simulink model "SF038A_LimrCdng"  (R2013b)
settings: Solver=FixedStepDiscrete  StartTime=0.0  StopTime=1  FixedStep=.002  RelTol=1e-3
values from neighbouring files (symbols this model uses):
  ARCHGLBPRM_2MILLISEC_SEC_F32 = DataDict.Constant    [SF038A_LimrCdng_DataDict.m]
  FLTINJ_LIMRCDNG_EOTGAIN = DataDict.Constant    [SF038A_LimrCdng_DataDict.m]
  FLTINJ_LIMRCDNG_EOTLIM = DataDict.Constant    [SF038A_LimrCdng_DataDict.m]
  FLTINJ_LIMRCDNG_SYSMOTTQCMDSCA = DataDict.Constant    [SF038A_LimrCdng_DataDict.m]
  LimrCdngGainDecSlew = DataDict.Calibration    [SF038A_LimrCdng_DataDict.m]
  LimrCdngTqDecSlew = DataDict.Calibration    [SF038A_LimrCdng_DataDict.m]
libraries: NxtrLim x12, FixdToFloat x2, LnrIntrpn x2, FloatToFixd x1, simulink x1
Description:
  | This function provides a layer of protection from erroneous signals feeding into SF-04 Sum & Limit.
  | It is applied primarily to 'limiting' signals that serve to reduce motor torque command under certain
  | operating conditions.  This function can prevent step response or 'toggling' behavior that might cause
  | undesirable vehicle feel.  It includes capability of fault injection at some inputs to facilitate tuning.
settings Model: CovMetricSettings=dcmw  CovHTMLOptions=-sRT=1 -aTS=1 -bRG=1 -bTC=1 -hTR=0 -nFC=0 -scm=1 -bcm=1 -xEv=0  Creator=Kevin Derry  LastModifiedBy=bzhf94
settings Model: ModifiedHistory=|
  | 001
  | Initial release
  | Kevin Derry
  | 15-Aug-2012
  | ICR-3666
  | 
  | 002
  | Add vehicle speed dependency to rate limiter cals applied during recovery (increasing direction).
  | Rename and share cals among rate limiters.
  | Scott Millsap
  | 14-May-2013
  | ICR-4115
  | 
  | 003
  | Added new input CCL_TrqRamp_Uls, a torque scaling factor calculated in the MSA function, and a rate limiter to limit the rate at which it changes.
  | Added new calibration to adjust the decreasing slew rate for CCL_TrqRamp_Uls.
  | Prerit Pramod
  | 09-July-2013
  | ICR-4202
  | 
  | 4.0.0
  | Updated Model according to the new FDD standards and tool chain.
  | Siva
  | 04-Feb-2015
  | ICR-XXXX
settings DataIOCC: LimitDataPoints=off  SaveFormat=Structure  ReturnWorkspaceOutputs=on
settings OptimizationCC: BlockReduction=off  InlineParams=on  ZeroExternalMemoryAtStartup=off  ZeroInternalMemoryAtStartup=off  OptimizeModelRefInitCode=on  LifeSpan=1
settings DebuggingCC: SignalInfNanChecking=error  SignalRangeChecking=warning  UnderspecifiedInitializationDetection=Simplified  SolverPrmCheckMsg=error  InheritedTsInSrcMsg=error  DiscreteInheritContinuousMsg=error  SingleTaskRateTransMsg=error  TasksWithSamePriorityMsg=error  SigSpecEnsureSampleTimeMsg=error  CheckMatrixSingularityMsg=error  IntegerOverflowMsg=error  ParameterUnderflowMsg=error  ParameterPrecisionLossMsg=error  ParameterTunabilityLossMsg=error  FixptConstUnderflowMsg=warning  FixptConstOverflowMsg=warning  VectorMatrixConversionMsg=error  SignalLabelMismatchMsg=error  UnconnectedInputMsg=error  UnconnectedOutputMsg=error  UnconnectedLineMsg=error  SFcnCompatibilityMsg=error  UniqueDataStoreMsg=warning  BusObjectLabelMismatch=error  RootOutportRequireBusObject=error  AssertControl=DisableAll  ModelReferenceIOMsg=error  ModelReferenceVersionMismatchMessage=warning  ModelReferenceIOMismatchMessage=error  ModelReferenceCSMismatchMessage=warning  ModelReferenceDataLoggingMessage=error  StateNameClashWarn=warning  StrictBusMsg=ErrorOnBusTreatedAsVector  NonBusSignalsTreatedAsBus=error  SFUnexpectedBacktrackingDiag=error  SFInvalidInputDataAccessInChartInitDiag=error  SFNoUnconditionalDefaultTransitionDiag=error  SFTransitionOutsideNaturalParentDiag=error  SFUnconditionalTransitionShadowingDiag=error  SFUndirectedBroadcastEventsDiag=error
settings ModelReferenceCC: ModelReferenceNumInstancesAllowed=Single
settings RTWCC: SystemTargetFile=autosar.tlc  GenCodeOnly=on  TemplateMakefile=ert_default_tmf  Description=AUTOSAR  GenerateReport=on  ProcessScript=autosar_make_rtw_hook  LaunchReport=on
settings CodeAppCC: GenerateComments=off  IgnoreCustomStorageClasses=off  CustomSymbolStrType=$N$R$M  CustomSymbolStrBlkIO=$N$M  SimulinkBlockComments=off
settings STFCustomTargetCC: ParMdlRefBuildCompliant=on  CompOptLevelCompliant=on  IncludeMdlTerminateFcn=off  CombineOutputUpdateFcns=on  SuppressErrorStatus=on  ERTFirstTimeCompliant=on  ERTCustomFileBanners=on  SupportNonFinite=off  SupportComplex=off  SupportContinuousTime=off  SupportNonInlinedSFcns=off  MATLABClassNameForMDSCustomization=Simulink.SoftwareTarget.ERTCustomization  AutosarCompliant=on  GRTInterface=off  SystemTargetFile=autosar.tlc
settings ERTTargetCC: CodeReplacementLibrary=ANSI_C  ConcurrentExecutionCompliant=off  IncludeMdlTerminateFcn=off  SuppressErrorStatus=on  SupportNonFinite=off  SupportComplex=off  ModelStepFunctionPrototypeControlCompliant=off  CPPClassGenCompliant=off  AutosarCompliant=on  InlinedParameterPlacement=NonHierarchical  ERTCustomFileTemplate=example_file_process.tlc  EnableUserReplacementTypes=on

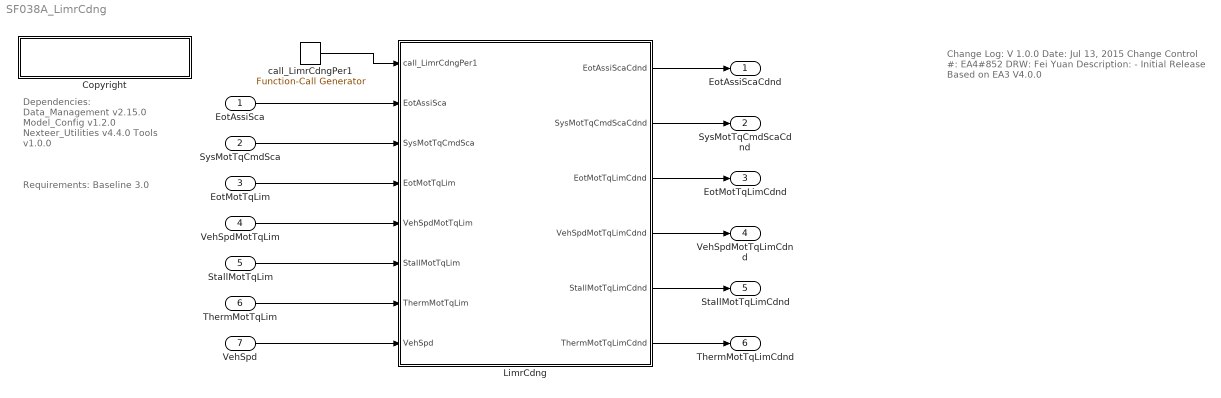
== system SF038A_LimrCdng ==
  note: Requirements: Baseline 3.0
  note: Dependencies:
      |   Data_Management v2.15.0
      |   Model_Config v1.2.0
      |   Nexteer_Utilities v4.4.0
      |   Tools v1.0.0
  note: Change Log:
      |
      | V 1.0.0
      | Date: Jul 13, 2015
      | Change Control #: EA4#852
      | DRW: Fei Yuan
      | Description:
      | - Initial Release Based on EA3 V4.0.0
  EotAssiSca : Inport
  SysMotTqCmdSca : Inport  Port=2
  EotMotTqLim : Inport  Port=3
  VehSpdMotTqLim : Inport  Port=4
  StallMotTqLim : Inport  Port=5
  ThermMotTqLim : Inport  Port=6
  VehSpd : Inport  Port=7
  Copyright : Subsystem  Description=|  mask(Copyright Information){none=on}
      | Copyright info block.                                               
      |                                                                     
      | Place copyright information at the top of every subsystem in design.
      mask prompts: none "No parameters"
      mask help: Place copyright information at the top of every subsystem in design.
      mask Display:
      | NxtrConf = 'Nexteer Confidential';
      | 
      | sys = bdroot; %handle for the current model ("system")
      | first = get_param(sys,'Created');
      | first = first(end-3:end);  %year is last four digits
      | 
      | last = get_param(sys,'LastModifiedDate');
      | if isempty(last)
      |     last = datestr(now,'yyyy');
      | else
      |     last = last(end-3:end);
      | end
      | 
      | if strcmp(first,last)
      |     fprintf('%s\nCopyright  %s Nexteer',NxtrConf,first);
      | else
      |     fprintf('%s\n%s%s-%s Nexteer',NxtrConf,char(169),first,last);
      | end
  LimrCdng : Subsystem
  call_LimrCdngPer1 : simulink/Ports & Subsystems/Function-Call Generator  RequirementInfo="{'linktype_rmi_doors' '0000a53e (/E-STEER Core/SubSystem Specifications/Application Functions/SF038A Limiter Conditioning)' '#SF038A_52' 'true' 'REQ:  SF038A_52' '' } %GIDa_33899db9_96af_4043_bf12_1f8199c4a9fb"  sample_time=0.002  numberOfIterations=1
      settings: AttributesFormatString=%<sample_time>
  EotAssiScaCdnd : Outport
  SysMotTqCmdScaCdnd : Outport  Port=2
  EotMotTqLimCdnd : Outport  Port=3
  VehSpdMotTqLimCdnd : Outport  Port=4
  StallMotTqLimCdnd : Outport  Port=5
  ThermMotTqLimCdnd : Outport  Port=6
  wires:
  call_LimrCdngPer1/1 -> LimrCdng/1(call_LimrCdngPer1)
  LimrCdng/3(EotMotTqLimCdnd) -> EotMotTqLimCdnd/1
  LimrCdng/4(VehSpdMotTqLimCdnd) -> VehSpdMotTqLimCdnd/1
  LimrCdng/5(StallMotTqLimCdnd) -> StallMotTqLimCdnd/1
  LimrCdng/6(ThermMotTqLimCdnd) -> ThermMotTqLimCdnd/1
  LimrCdng/2(SysMotTqCmdScaCdnd) -> SysMotTqCmdScaCdnd/1
  LimrCdng/1(EotAssiScaCdnd) -> EotAssiScaCdnd/1
  VehSpdMotTqLim/1 -> LimrCdng/5(VehSpdMotTqLim)
  ThermMotTqLim/1 -> LimrCdng/7(ThermMotTqLim)
  SysMotTqCmdSca/1 -> LimrCdng/3(SysMotTqCmdSca)
  EotMotTqLim/1 -> LimrCdng/4(EotMotTqLim)
  EotAssiSca/1 -> LimrCdng/2(EotAssiSca)
  StallMotTqLim/1 -> LimrCdng/6(StallMotTqLim)
  VehSpd/1 -> LimrCdng/8(VehSpd)

== system SF038A_LimrCdng/Copyright ==

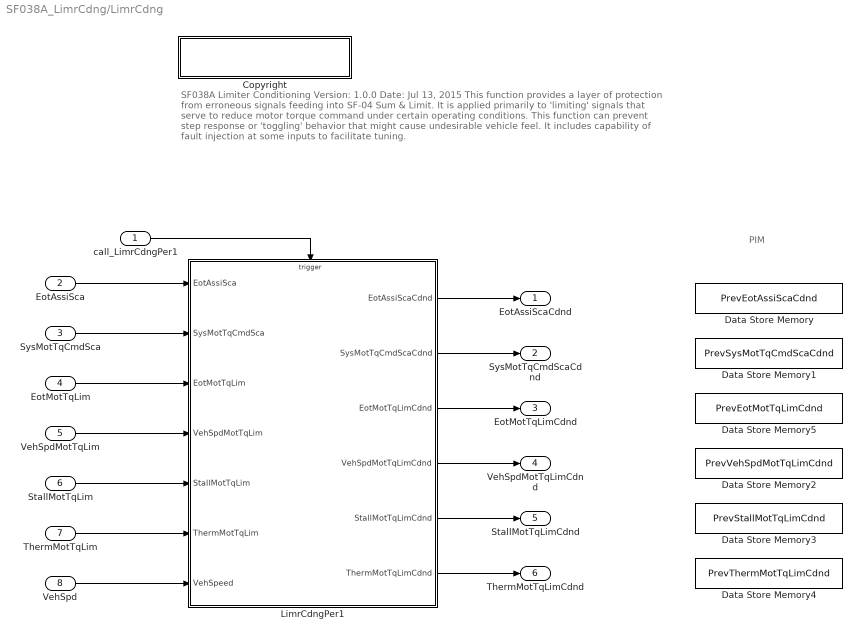
== system SF038A_LimrCdng/LimrCdng ==
  note: PIM
  note: SF038A  Limiter Conditioning
      | Version:  1.0.0     Date:  Jul 13, 2015
      |
      | This function provides a layer of protection from erroneous signals feeding into SF-04 Sum & Limit.
      | It is applied primarily to 'limiting' signals that serve to reduce motor torque command under certain
      | operating conditions.  This function can prevent step response or 'toggling' behavior that might cause
      | undesirable vehicle feel.  It includes capability of fault injection at some inputs to facilitate tuning.
  call_LimrCdngPer1 : Inport
  EotAssiSca : Inport  RequirementInfo="{'linktype_rmi_doors' '0000a53e (/E-STEER Core/SubSystem Specifications/Application Functions/SF038A Limiter Conditioning)' '#SF038A_9' 'true' 'REQ:  SF038A_9' '' } %GIDa_95b6a5c9_0ea2_4b71_a18e_8af6141b721d"  Port=2
  SysMotTqCmdSca : Inport  RequirementInfo="{'linktype_rmi_doors' '0000a53e (/E-STEER Core/SubSystem Specifications/Application Functions/SF038A Limiter Conditioning)' '#SF038A_32' 'true' 'REQ:  SF038A_32' '' } %GIDa_d644cb2e_06c7_46bd_9f8c_2e58e9e11dd4"  Port=3
  EotMotTqLim : Inport  RequirementInfo="{'linktype_rmi_doors' '0000a53e (/E-STEER Core/SubSystem Specifications/Application Functions/SF038A Limiter Conditioning)' '#SF038A_33' 'true' 'REQ:  SF038A_33' '' } %GIDa_34eaac59_c46a_4a86_98aa_7316f8ddc777"  Port=4
  VehSpdMotTqLim : Inport  RequirementInfo="{'linktype_rmi_doors' '0000a53e (/E-STEER Core/SubSystem Specifications/Application Functions/SF038A Limiter Conditioning)' '#SF038A_34' 'true' 'REQ:  SF038A_34' '' } %GIDa_5871f326_e5eb_4bf5_971f_60224a1642be"  Port=5
  StallMotTqLim : Inport  RequirementInfo="{'linktype_rmi_doors' '0000a53e (/E-STEER Core/SubSystem Specifications/Application Functions/SF038A Limiter Conditioning)' '#SF038A_35' 'true' 'REQ:  SF038A_35' '' } %GIDa_b9e54dce_09d0_4883_abfa_7d2a02c8cade"  Port=6
  ThermMotTqLim : Inport  RequirementInfo="{'linktype_rmi_doors' '0000a53e (/E-STEER Core/SubSystem Specifications/Application Functions/SF038A Limiter Conditioning)' '#SF038A_36' 'true' 'REQ:  SF038A_36' '' } %GIDa_e62a3544_49ac_4587_8d34_9b4d1dff1da3"  Port=7
  VehSpd : Inport  RequirementInfo="{'linktype_rmi_doors' '0000a53e (/E-STEER Core/SubSystem Specifications/Application Functions/SF038A Limiter Conditioning)' '#SF038A_37' 'true' 'REQ:  SF038A_37' '' } %GIDa_20705676_3852_4d53_b159_210d5e5d8ae2"  Port=8
  Copyright : Subsystem  Description=|  mask(Copyright Information){none=on}
      | Copyright info block.                                               
      |                                                                     
      | Place copyright information at the top of every subsystem in design.
      mask prompts: none "No parameters"
      mask help: Place copyright information at the top of every subsystem in design.
      mask Display:
      | NxtrConf = 'Nexteer Confidential';
      | 
      | sys = bdroot; %handle for the current model ("system")
      | first = get_param(sys,'Created');
      | first = first(end-3:end);  %year is last four digits
      | 
      | last = get_param(sys,'LastModifiedDate');
      | if isempty(last)
      |     last = datestr(now,'yyyy');
      | else
      |     last = last(end-3:end);
      | end
      | 
      | if strcmp(first,last)
      |     fprintf('%s\nCopyright  %s Nexteer',NxtrConf,first);
      | else
      |     fprintf('%s\n%s%s-%s Nexteer',NxtrConf,char(169),first,last);
      | end
  Data Store Memory : DataStoreMemory  DataStoreName=PrevEotAssiScaCdnd  StateMustResolveToSignalObject=on
  Data Store Memory1 : DataStoreMemory  DataStoreName=PrevSysMotTqCmdScaCdnd  StateMustResolveToSignalObject=on
  Data Store Memory2 : DataStoreMemory  DataStoreName=PrevVehSpdMotTqLimCdnd  StateMustResolveToSignalObject=on
  Data Store Memory3 : DataStoreMemory  DataStoreName=PrevStallMotTqLimCdnd  StateMustResolveToSignalObject=on
  Data Store Memory4 : DataStoreMemory  DataStoreName=PrevThermMotTqLimCdnd  StateMustResolveToSignalObject=on
  Data Store Memory5 : DataStoreMemory  DataStoreName=PrevEotMotTqLimCdnd  StateMustResolveToSignalObject=on
  LimrCdngPer1 : Subsystem
  EotAssiScaCdnd : Outport  RequirementInfo="{'linktype_rmi_doors' '0000a53e (/E-STEER Core/SubSystem Specifications/Application Functions/SF038A Limiter Conditioning)' '#SF038A_11' 'true' 'REQ:  SF038A_11' '' } %GIDa_ad921279_63de_4e0a_b9d8_ae490232194c"
  SysMotTqCmdScaCdnd : Outport  RequirementInfo="{'linktype_rmi_doors' '0000a53e (/E-STEER Core/SubSystem Specifications/Application Functions/SF038A Limiter Conditioning)' '#SF038A_39' 'true' 'REQ:  SF038A_39' '' } %GIDa_479dd64d_355a_424c_9143_244779bf715c"  Port=2
  EotMotTqLimCdnd : Outport  RequirementInfo="{'linktype_rmi_doors' '0000a53e (/E-STEER Core/SubSystem Specifications/Application Functions/SF038A Limiter Conditioning)' '#SF038A_40' 'true' 'REQ:  SF038A_40' '' } %GIDa_d35a5d0a_1d3f_4b4d_a2f7_876f98b59f29"  Port=3
  VehSpdMotTqLimCdnd : Outport  RequirementInfo="{'linktype_rmi_doors' '0000a53e (/E-STEER Core/SubSystem Specifications/Application Functions/SF038A Limiter Conditioning)' '#SF038A_41' 'true' 'REQ:  SF038A_41' '' } %GIDa_fa7d0305_147a_4137_9a13_a989878fb15c"  Port=4
  StallMotTqLimCdnd : Outport  RequirementInfo="{'linktype_rmi_doors' '0000a53e (/E-STEER Core/SubSystem Specifications/Application Functions/SF038A Limiter Conditioning)' '#SF038A_42' 'true' 'REQ:  SF038A_42' '' } %GIDa_e84169d6_dc44_4223_a409_313b28b2f464"  Port=5
  ThermMotTqLimCdnd : Outport  RequirementInfo="{'linktype_rmi_doors' '0000a53e (/E-STEER Core/SubSystem Specifications/Application Functions/SF038A Limiter Conditioning)' '#SF038A_43' 'true' 'REQ:  SF038A_43' '' } %GIDa_8885543d_4d63_4528_a500_fb56e7e71977"  Port=6
  wires:
  LimrCdngPer1/1(EotAssiScaCdnd) -> EotAssiScaCdnd/1
  LimrCdngPer1/2(SysMotTqCmdScaCdnd) -> SysMotTqCmdScaCdnd/1
  LimrCdngPer1/3(EotMotTqLimCdnd) -> EotMotTqLimCdnd/1
  LimrCdngPer1/4(VehSpdMotTqLimCdnd) -> VehSpdMotTqLimCdnd/1
  LimrCdngPer1/5(StallMotTqLimCdnd) -> StallMotTqLimCdnd/1
  LimrCdngPer1/6(ThermMotTqLimCdnd) -> ThermMotTqLimCdnd/1
  call_LimrCdngPer1/1 -> LimrCdngPer1/Trigger
  EotAssiSca/1 -> LimrCdngPer1/1(EotAssiSca)
  SysMotTqCmdSca/1 -> LimrCdngPer1/2(SysMotTqCmdSca)
  EotMotTqLim/1 -> LimrCdngPer1/3(EotMotTqLim)
  VehSpdMotTqLim/1 -> LimrCdngPer1/4(VehSpdMotTqLim)
  StallMotTqLim/1 -> LimrCdngPer1/5(StallMotTqLim)
  ThermMotTqLim/1 -> LimrCdngPer1/6(ThermMotTqLim)
  VehSpd/1 -> LimrCdngPer1/7(VehSpeed)

== system SF038A_LimrCdng/LimrCdng/Copyright ==

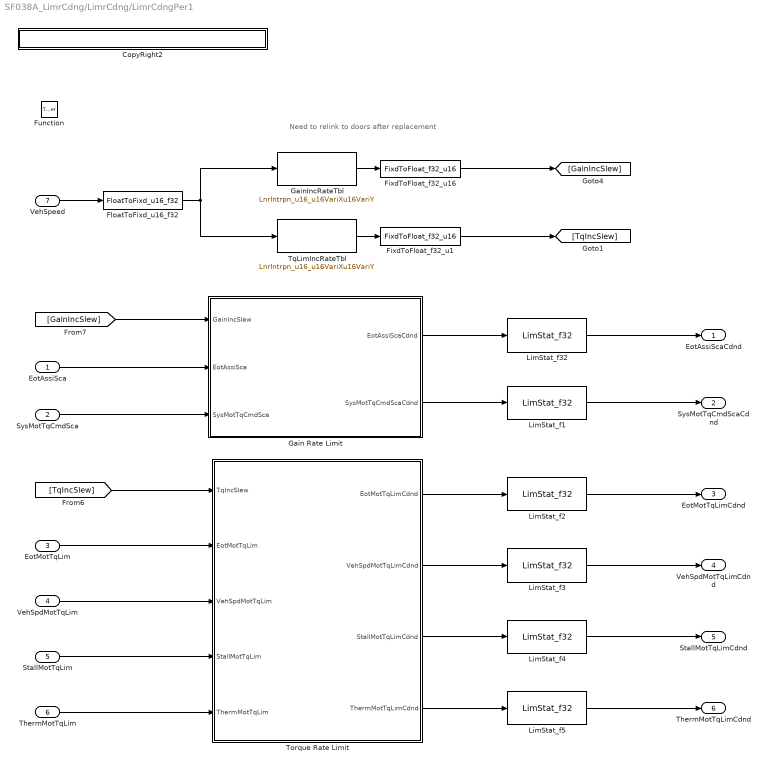
== system SF038A_LimrCdng/LimrCdng/LimrCdngPer1 ==
  note: Need to relink to doors after replacement
  EotAssiSca : Inport
  SysMotTqCmdSca : Inport  Port=2
  EotMotTqLim : Inport  Port=3
  VehSpdMotTqLim : Inport  Port=4
  StallMotTqLim : Inport  Port=5
  ThermMotTqLim : Inport  Port=6
  VehSpeed : Inport  Port=7
  Function : TriggerPort  TriggerType=function-call  PortDimensions=1
  CopyRight2 : Subsystem  Description=|  mask(Copyright Information){none=on}
      | Copyright info block.                                               
      |                                                                     
      | Place copyright information at the top of every subsystem in design.
      mask prompts: none "No parameters"
      mask help: Place copyright information at the top of every subsystem in design.
      mask Display:
      | NxtrConf = 'Nexteer Confidential';
      | 
      | sys = bdroot; %handle for the current model ("system")
      | first = get_param(sys,'Created');
      | first = first(end-3:end);  %year is last four digits
      | 
      | last = get_param(sys,'LastModifiedDate');
      | if isempty(last)
      |     last = datestr(now,'yyyy');
      | else
      |     last = last(end-3:end);
      | end
      | 
      | if strcmp(first,last)
      |     fprintf('%s -- Copyright %s Nexteer',NxtrConf,first)
      | else
      |     fprintf('%s -- %s%s- %s Nexteer',NxtrConf,char(169),first,last)
      | end
  FixdToFloat_f32_u1 : FixdToFloat/FixdToFloat_f32_u16  Param1=3
  FixdToFloat_f32_u16 : FixdToFloat/FixdToFloat_f32_u16  Param1=7
  FloatToFixd_u16_f32 : FloatToFixd/FloatToFixd_u16_f32  Param1=7
  Gain Rate Limit : Subsystem  RequirementInfo={} %GIDa_e7594f3f_ee15_4243_8876_6805bb8800ba
  GainIncRateTbl : LnrIntrpn/LnrIntrpn_u16_u16VariXu16VariY  RequirementInfo="{'linktype_rmi_doors' '0000a53e (/E-STEER Core/SubSystem Specifications/Application Functions/SF038A Limiter Conditioning)' '#SF038A_62' 'true' 'REQ:  SF038A_62' '' ; 'linktype_rmi_doors' '0000a53e (/E-STEER Core/SubSystem Specifications/Application Functions/SF038A Limiter Conditioning)' '#SF038A_83' 'true' 'REQ:  SF038A_83' '' } %GIDa_d2538397_2c5f_48ed_9b0c_63955ca9bdcf"  XTbl=LimrCdngGainIncSlewX  YTbl=LimrCdngGainIncSlewY
      settings: AttributesFormatString=Lnr ( u16VariX , u16VariY )
  LimStat_f1 : NxtrLim/LimStat_f32  RequirementInfo="{'linktype_rmi_doors' '0000a53e (/E-STEER Core/SubSystem Specifications/Application Functions/SF038A Limiter Conditioning)' '#SF038A_87' 'true' 'REQ:  SF038A_87' '' } %GIDa_7d845a5a_348d_44d3_9cc0_de7506ae8106"  LoLim=GAINLOLIM_ULS_F32  HiLim=GAINHILIM_ULS_F32
      settings: AttributesFormatString=|
      | Low Limit: %<LoLim>
      | High Limit:%<HiLim>
  LimStat_f2 : NxtrLim/LimStat_f32  RequirementInfo="{'linktype_rmi_doors' '0000a53e (/E-STEER Core/SubSystem Specifications/Application Functions/SF038A Limiter Conditioning)' '#SF038A_88' 'true' 'REQ:  SF038A_88' '' } %GIDa_92372c16_e6a8_438c_9999_908ed739753b"  LoLim=MOTTQLOLIMCDNG_MOTNWTMTR_F32  HiLim=SYSGLBPRM_MOTTQCMDHILIM_MOTNWTMTR_F32
      settings: AttributesFormatString=|
      | Low Limit: %<LoLim>
      | High Limit:%<HiLim>
  LimStat_f3 : NxtrLim/LimStat_f32  RequirementInfo="{'linktype_rmi_doors' '0000a53e (/E-STEER Core/SubSystem Specifications/Application Functions/SF038A Limiter Conditioning)' '#SF038A_88' 'true' 'REQ:  SF038A_88' '' } %GIDa_238f40fa_f8e2_4483_b79a_2126bca3690f"  LoLim=MOTTQLOLIMCDNG_MOTNWTMTR_F32  HiLim=SYSGLBPRM_MOTTQCMDHILIM_MOTNWTMTR_F32
      settings: AttributesFormatString=|
      | Low Limit: %<LoLim>
      | High Limit:%<HiLim>
  LimStat_f32 : NxtrLim/LimStat_f32  RequirementInfo="{'linktype_rmi_doors' '0000a53e (/E-STEER Core/SubSystem Specifications/Application Functions/SF038A Limiter Conditioning)' '#SF038A_87' 'true' 'REQ:  SF038A_87' '' } %GIDa_c7e369cd_abd8_4804_8058_36b2eef7c18f"  LoLim=GAINLOLIM_ULS_F32  HiLim=GAINHILIM_ULS_F32
      settings: AttributesFormatString=|
      | Low Limit: %<LoLim>
      | High Limit:%<HiLim>
  LimStat_f4 : NxtrLim/LimStat_f32  RequirementInfo="{'linktype_rmi_doors' '0000a53e (/E-STEER Core/SubSystem Specifications/Application Functions/SF038A Limiter Conditioning)' '#SF038A_88' 'true' 'REQ:  SF038A_88' '' } %GIDa_8a1c0711_c956_4289_aa20_982859c8e232"  LoLim=MOTTQLOLIMCDNG_MOTNWTMTR_F32  HiLim=SYSGLBPRM_MOTTQCMDHILIM_MOTNWTMTR_F32
      settings: AttributesFormatString=|
      | Low Limit: %<LoLim>
      | High Limit:%<HiLim>
  LimStat_f5 : NxtrLim/LimStat_f32  RequirementInfo="{'linktype_rmi_doors' '0000a53e (/E-STEER Core/SubSystem Specifications/Application Functions/SF038A Limiter Conditioning)' '#SF038A_88' 'true' 'REQ:  SF038A_88' '' } %GIDa_2cc05737_5cdd_491a_87ed_dc6d3ffe7604"  LoLim=MOTTQLOLIMCDNG_MOTNWTMTR_F32  HiLim=SYSGLBPRM_MOTTQCMDHILIM_MOTNWTMTR_F32
      settings: AttributesFormatString=|
      | Low Limit: %<LoLim>
      | High Limit:%<HiLim>
  Torque Rate Limit : Subsystem  RequirementInfo={} %GIDa_7b36ccd2_790b_4668_ad54_781e7693bf1b
  TqLimIncRateTbl : LnrIntrpn/LnrIntrpn_u16_u16VariXu16VariY  RequirementInfo="{'linktype_rmi_doors' '0000a53e (/E-STEER Core/SubSystem Specifications/Application Functions/SF038A Limiter Conditioning)' '#SF038A_84' 'true' 'REQ:  SF038A_84' '' ; 'linktype_rmi_doors' '0000a53e (/E-STEER Core/SubSystem Specifications/Application Functions/SF038A Limiter Conditioning)' '#SF038A_83' 'true' 'REQ:  SF038A_83' '' } %GIDa_69585301_2513_4152_803c_7030eb8e14c5"  XTbl=LimrCdngTqIncSlewX  YTbl=LimrCdngTqIncSlewY
      settings: AttributesFormatString=Lnr ( u16VariX , u16VariY )
  EotAssiScaCdnd : Outport
  SysMotTqCmdScaCdnd : Outport  Port=2
  EotMotTqLimCdnd : Outport  Port=3
  VehSpdMotTqLimCdnd : Outport  Port=4
  StallMotTqLimCdnd : Outport  Port=5
  ThermMotTqLimCdnd : Outport  Port=6
  wires:
  VehSpeed/1 -> FloatToFixd_u16_f32/1
  GainIncRateTbl/1 -> FixdToFloat_f32_u16/1
  TqLimIncRateTbl/1 -> FixdToFloat_f32_u1/1
  EotMotTqLim/1 -> Torque Rate Limit/2(EotMotTqLim)
  VehSpdMotTqLim/1 -> Torque Rate Limit/3(VehSpdMotTqLim)
  StallMotTqLim/1 -> Torque Rate Limit/4(StallMotTqLim)
  ThermMotTqLim/1 -> Torque Rate Limit/5(ThermMotTqLim)
  Torque Rate Limit/1(EotMotTqLimCdnd) -> LimStat_f2/1
  Torque Rate Limit/2(VehSpdMotTqLimCdnd) -> LimStat_f3/1
  Torque Rate Limit/3(StallMotTqLimCdnd) -> LimStat_f4/1
  Torque Rate Limit/4(ThermMotTqLimCdnd) -> LimStat_f5/1
  [TqIncSlew] -> Torque Rate Limit/1(TqIncSlew)
  EotAssiSca/1 -> Gain Rate Limit/2(EotAssiSca)
  SysMotTqCmdSca/1 -> Gain Rate Limit/3(SysMotTqCmdSca)
  Gain Rate Limit/1(EotAssiScaCdnd) -> LimStat_f32/1
  Gain Rate Limit/2(SysMotTqCmdScaCdnd) -> LimStat_f1/1
  [GainIncSlew] -> Gain Rate Limit/1(GainIncSlew)
  FloatToFixd_u16_f32/1 -> TqLimIncRateTbl/1, GainIncRateTbl/1
  FixdToFloat_f32_u16/1 -> [GainIncSlew]
  FixdToFloat_f32_u1/1 -> [TqIncSlew]
  LimStat_f32/1 -> EotAssiScaCdnd/1
  LimStat_f1/1 -> SysMotTqCmdScaCdnd/1
  LimStat_f2/1 -> EotMotTqLimCdnd/1
  LimStat_f3/1 -> VehSpdMotTqLimCdnd/1
  LimStat_f4/1 -> StallMotTqLimCdnd/1
  LimStat_f5/1 -> ThermMotTqLimCdnd/1

== system SF038A_LimrCdng/LimrCdng/LimrCdngPer1/CopyRight2 ==

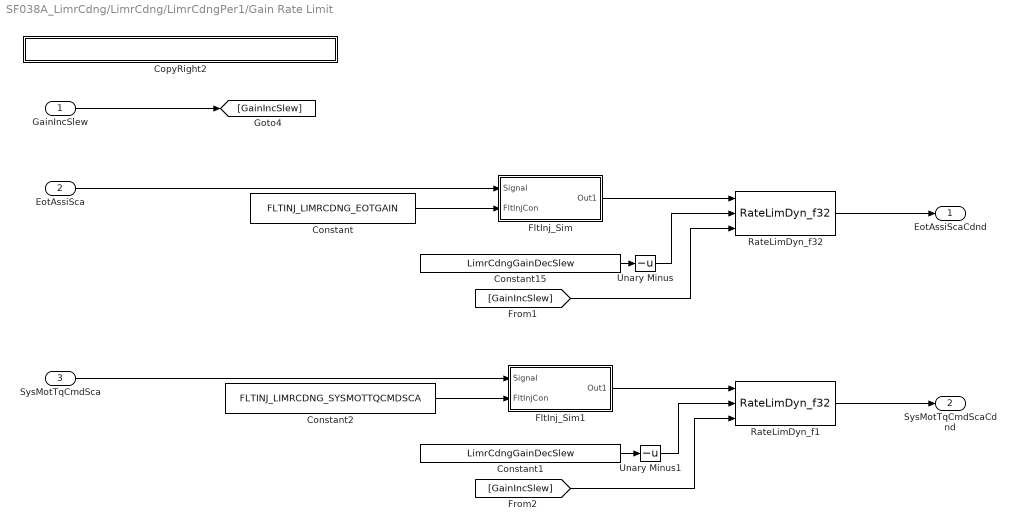
== system SF038A_LimrCdng/LimrCdng/LimrCdngPer1/Gain Rate Limit ==
  GainIncSlew : Inport
  EotAssiSca : Inport  Port=2
  SysMotTqCmdSca : Inport  Port=3
  Constant : Constant  Value=FLTINJ_LIMRCDNG_EOTGAIN
  Constant1 : Constant  RequirementInfo="{'linktype_rmi_doors' '0000a53e (/E-STEER Core/SubSystem Specifications/Application Functions/SF038A Limiter Conditioning)' '#SF038A_90' 'true' 'REQ:  SF038A_90' '' } %GIDa_c1cd19f4_dc05_4fef_976b_df920917e707"  Value=LimrCdngGainDecSlew
  Constant15 : Constant  RequirementInfo="{'linktype_rmi_doors' '0000a53e (/E-STEER Core/SubSystem Specifications/Application Functions/SF038A Limiter Conditioning)' '#SF038A_90' 'true' 'REQ:  SF038A_90' '' } %GIDa_0a260758_1920_4a6f_b2fa_f6b6932bbd19"  Value=LimrCdngGainDecSlew
  Constant2 : Constant  Value=FLTINJ_LIMRCDNG_SYSMOTTQCMDSCA
  CopyRight2 : Subsystem  Description=|  mask(Copyright Information){none=on}
      | Copyright info block.                                               
      |                                                                     
      | Place copyright information at the top of every subsystem in design.
      mask prompts: none "No parameters"
      mask help: Place copyright information at the top of every subsystem in design.
      mask Display:
      | NxtrConf = 'Nexteer Confidential';
      | 
      | sys = bdroot; %handle for the current model ("system")
      | first = get_param(sys,'Created');
      | first = first(end-3:end);  %year is last four digits
      | 
      | last = get_param(sys,'LastModifiedDate');
      | if isempty(last)
      |     last = datestr(now,'yyyy');
      | else
      |     last = last(end-3:end);
      | end
      | 
      | if strcmp(first,last)
      |     fprintf('%s -- Copyright %s Nexteer',NxtrConf,first)
      | else
      |     fprintf('%s -- %s%s- %s Nexteer',NxtrConf,char(169),first,last)
      | end
  FltInj_Sim : Subsystem  RequirementInfo="{'linktype_rmi_doors' '0000a53e (/E-STEER Core/SubSystem Specifications/Application Functions/SF038A Limiter Conditioning)' '#SF038A_74' 'true' 'REQ:  SF038A_74' '' } %GIDa_935a8007_ab29_4aec_9ca4_6cf65bf5bb28"  TreatAsAtomicUnit=on  VariantControl=FltInj_sim  mask(Fault_Injection){}
      mask help: Fault Injection is a simulation only block for EA4 programs.
  FltInj_Sim1 : Subsystem  RequirementInfo="{'linktype_rmi_doors' '0000a53e (/E-STEER Core/SubSystem Specifications/Application Functions/SF038A Limiter Conditioning)' '#SF038A_75' 'true' 'REQ:  SF038A_75' '' } %GIDa_8e7db811_7c34_4c11_baa8_f817e058618e"  TreatAsAtomicUnit=on  VariantControl=FltInj_sim  mask(Fault_Injection){}
      mask help: Fault Injection is a simulation only block for EA4 programs.
  RateLimDyn_f1 : NxtrLim/RateLimDyn_f32  RequirementInfo="{'linktype_rmi_doors' '0000a53e (/E-STEER Core/SubSystem Specifications/Application Functions/SF038A Limiter Conditioning)' '#SF038A_68' 'true' 'REQ:  SF038A_68' '' } %GIDa_c6803a6f_0b4b_4041_b73e_45209b9f107c"  StVar=PrevSysMotTqCmdScaCdnd  Ts=ARCHGLBPRM_2MILLISEC_SEC_F32
      settings: AttributesFormatString=StVar: %<StVar>
  RateLimDyn_f32 : NxtrLim/RateLimDyn_f32  RequirementInfo="{'linktype_rmi_doors' '0000a53e (/E-STEER Core/SubSystem Specifications/Application Functions/SF038A Limiter Conditioning)' '#SF038A_68' 'true' 'REQ:  SF038A_68' '' } %GIDa_9623ec69_d93e_48de_9a57_55355c7f5f10"  StVar=PrevEotAssiScaCdnd  Ts=ARCHGLBPRM_2MILLISEC_SEC_F32
      settings: AttributesFormatString=StVar: %<StVar>
  Unary Minus : UnaryMinus
  Unary Minus1 : UnaryMinus
  EotAssiScaCdnd : Outport
  SysMotTqCmdScaCdnd : Outport  Port=2
  wires:
  [GainIncSlew] -> RateLimDyn_f32/3
  FltInj_Sim/1(Out1) -> RateLimDyn_f32/1
  Unary Minus/1 -> RateLimDyn_f32/2
  Constant15/1 -> Unary Minus/1
  FltInj_Sim1/1(Out1) -> RateLimDyn_f1/1
  RateLimDyn_f1/1 -> SysMotTqCmdScaCdnd/1
  EotAssiSca/1 -> FltInj_Sim/1(Signal)
  RateLimDyn_f32/1 -> EotAssiScaCdnd/1
  GainIncSlew/1 -> [GainIncSlew]
  SysMotTqCmdSca/1 -> FltInj_Sim1/1(Signal)
  Constant1/1 -> Unary Minus1/1
  Unary Minus1/1 -> RateLimDyn_f1/2
  Constant/1 -> FltInj_Sim/2(FltInjCon)
  Constant2/1 -> FltInj_Sim1/2(FltInjCon)
  [GainIncSlew] -> RateLimDyn_f1/3

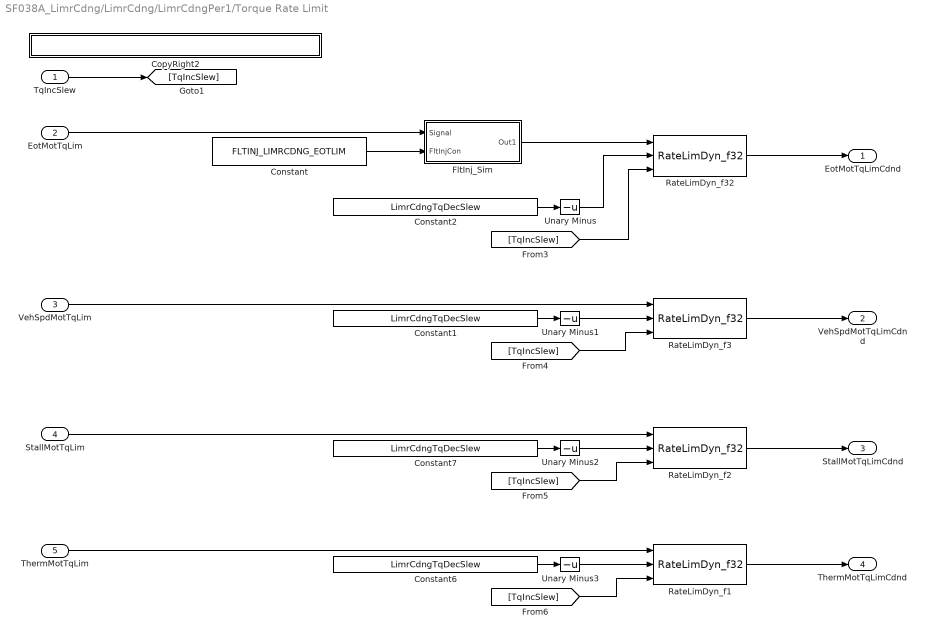
== system SF038A_LimrCdng/LimrCdng/LimrCdngPer1/Torque Rate Limit ==
  TqIncSlew : Inport
  EotMotTqLim : Inport  Port=2
  VehSpdMotTqLim : Inport  Port=3
  StallMotTqLim : Inport  Port=4
  ThermMotTqLim : Inport  Port=5
  Constant : Constant  Value=FLTINJ_LIMRCDNG_EOTLIM
  Constant1 : Constant  RequirementInfo="{'linktype_rmi_doors' '0000a53e (/E-STEER Core/SubSystem Specifications/Application Functions/SF038A Limiter Conditioning)' '#SF038A_91' 'true' 'REQ:  SF038A_91' '' } %GIDa_3a17f3b4_938f_48ba_9143_e2482409a21b"  Value=LimrCdngTqDecSlew
  Constant2 : Constant  RequirementInfo="{'linktype_rmi_doors' '0000a53e (/E-STEER Core/SubSystem Specifications/Application Functions/SF038A Limiter Conditioning)' '#SF038A_91' 'true' 'REQ:  SF038A_91' '' } %GIDa_04e30fea_239e_4531_90e1_4ffa78575852"  Value=LimrCdngTqDecSlew
  Constant6 : Constant  RequirementInfo="{'linktype_rmi_doors' '0000a53e (/E-STEER Core/SubSystem Specifications/Application Functions/SF038A Limiter Conditioning)' '#SF038A_91' 'true' 'REQ:  SF038A_91' '' } %GIDa_87b377d4_b336_44e5_955c_6b2f27b4dc47"  Value=LimrCdngTqDecSlew
  Constant7 : Constant  RequirementInfo="{'linktype_rmi_doors' '0000a53e (/E-STEER Core/SubSystem Specifications/Application Functions/SF038A Limiter Conditioning)' '#SF038A_91' 'true' 'REQ:  SF038A_91' '' } %GIDa_6d3e5583_cc5f_4b34_b101_cc44db36dd03"  Value=LimrCdngTqDecSlew
  CopyRight2 : Subsystem  Description=|  mask(Copyright Information){none=on}
      | Copyright info block.                                               
      |                                                                     
      | Place copyright information at the top of every subsystem in design.
      mask prompts: none "No parameters"
      mask help: Place copyright information at the top of every subsystem in design.
      mask Display:
      | NxtrConf = 'Nexteer Confidential';
      | 
      | sys = bdroot; %handle for the current model ("system")
      | first = get_param(sys,'Created');
      | first = first(end-3:end);  %year is last four digits
      | 
      | last = get_param(sys,'LastModifiedDate');
      | if isempty(last)
      |     last = datestr(now,'yyyy');
      | else
      |     last = last(end-3:end);
      | end
      | 
      | if strcmp(first,last)
      |     fprintf('%s -- Copyright %s Nexteer',NxtrConf,first)
      | else
      |     fprintf('%s -- %s%s- %s Nexteer',NxtrConf,char(169),first,last)
      | end
  FltInj_Sim : Subsystem  RequirementInfo="{'linktype_rmi_doors' '0000a53e (/E-STEER Core/SubSystem Specifications/Application Functions/SF038A Limiter Conditioning)' '#SF038A_76' 'true' 'REQ:  SF038A_76' '' } %GIDa_e310a8e9_57f2_4254_b9f9_cd45ce5ce9f1"  TreatAsAtomicUnit=on  VariantControl=FltInj_sim  mask(Fault_Injection){}
      mask help: Fault Injection is a simulation only block for EA4 programs.
  RateLimDyn_f1 : NxtrLim/RateLimDyn_f32  RequirementInfo="{'linktype_rmi_doors' '0000a53e (/E-STEER Core/SubSystem Specifications/Application Functions/SF038A Limiter Conditioning)' '#SF038A_72' 'true' 'REQ:  SF038A_72' '' } %GIDa_b21d8b69_6c39_43f2_9098_0bcedd6d7462"  StVar=PrevThermMotTqLimCdnd  Ts=ARCHGLBPRM_2MILLISEC_SEC_F32
      settings: AttributesFormatString=StVar: %<StVar>
  RateLimDyn_f2 : NxtrLim/RateLimDyn_f32  RequirementInfo="{'linktype_rmi_doors' '0000a53e (/E-STEER Core/SubSystem Specifications/Application Functions/SF038A Limiter Conditioning)' '#SF038A_72' 'true' 'REQ:  SF038A_72' '' } %GIDa_a45545b0_9d64_4bc5_82e4_20835f1f503f"  StVar=PrevStallMotTqLimCdnd  Ts=ARCHGLBPRM_2MILLISEC_SEC_F32
      settings: AttributesFormatString=StVar: %<StVar>
  RateLimDyn_f3 : NxtrLim/RateLimDyn_f32  RequirementInfo="{'linktype_rmi_doors' '0000a53e (/E-STEER Core/SubSystem Specifications/Application Functions/SF038A Limiter Conditioning)' '#SF038A_72' 'true' 'REQ:  SF038A_72' '' } %GIDa_50a34468_6712_4e81_903f_b971b061f3bf"  StVar=PrevVehSpdMotTqLimCdnd  Ts=ARCHGLBPRM_2MILLISEC_SEC_F32
      settings: AttributesFormatString=StVar: %<StVar>
  RateLimDyn_f32 : NxtrLim/RateLimDyn_f32  RequirementInfo="{'linktype_rmi_doors' '0000a53e (/E-STEER Core/SubSystem Specifications/Application Functions/SF038A Limiter Conditioning)' '#SF038A_72' 'true' 'REQ:  SF038A_72' '' } %GIDa_d8324b34_424c_4c99_b965_6f35754556d9"  StVar=PrevEotMotTqLimCdnd  Ts=ARCHGLBPRM_2MILLISEC_SEC_F32
      settings: AttributesFormatString=StVar: %<StVar>
  Unary Minus{,1..3} (4 alike) : UnaryMinus
  EotMotTqLimCdnd : Outport
  VehSpdMotTqLimCdnd : Outport  Port=2
  StallMotTqLimCdnd : Outport  Port=3
  ThermMotTqLimCdnd : Outport  Port=4
  wires:
  RateLimDyn_f2/1 -> StallMotTqLimCdnd/1
  RateLimDyn_f3/1 -> VehSpdMotTqLimCdnd/1
  Unary Minus3/1 -> RateLimDyn_f1/2
  RateLimDyn_f1/1 -> ThermMotTqLimCdnd/1
  RateLimDyn_f32/1 -> EotMotTqLimCdnd/1
  [TqIncSlew] -> RateLimDyn_f1/3
  Constant/1 -> FltInj_Sim/2(FltInjCon)
  Constant6/1 -> Unary Minus3/1
  Constant2/1 -> Unary Minus/1
  Unary Minus1/1 -> RateLimDyn_f3/2
  FltInj_Sim/1(Out1) -> RateLimDyn_f32/1
  Constant7/1 -> Unary Minus2/1
  Unary Minus2/1 -> RateLimDyn_f2/2
  Constant1/1 -> Unary Minus1/1
  Unary Minus/1 -> RateLimDyn_f32/2
  EotMotTqLim/1 -> FltInj_Sim/1(Signal)
  [TqIncSlew] -> RateLimDyn_f32/3
  [TqIncSlew] -> RateLimDyn_f3/3
  [TqIncSlew] -> RateLimDyn_f2/3
  TqIncSlew/1 -> [TqIncSlew]
  ThermMotTqLim/1 -> RateLimDyn_f1/1
  StallMotTqLim/1 -> RateLimDyn_f2/1
  VehSpdMotTqLim/1 -> RateLimDyn_f3/1

== system SF038A_LimrCdng/LimrCdng/LimrCdngPer1/Gain Rate Limit/CopyRight2 ==

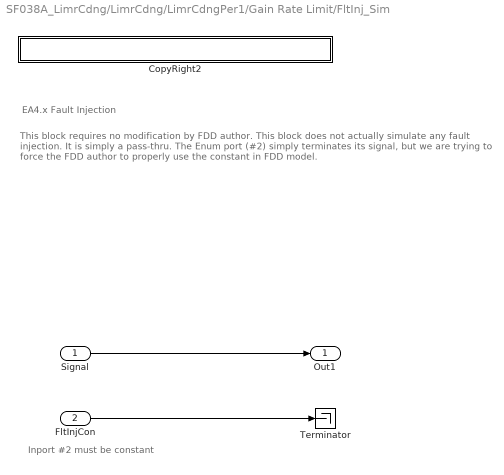
== system SF038A_LimrCdng/LimrCdng/LimrCdngPer1/Gain Rate Limit/FltInj_Sim ==
  note: This block requires no modification by FDD author.
      |
      | This block does not actually simulate any fault injection.  It is simply a pass-thru.
      |
      | The Enum port (#2) simply terminates its signal, but we are trying to force the FDD author
      | to properly use the constant in FDD model.
  note: EA4.x Fault Injection
  note: Inport #2 must be constant
  Signal : Inport
  FltInjCon : Inport  Port=2
  CopyRight2 : Subsystem  Description=|  mask(Copyright Information){none=on}
      | Copyright info block.                                               
      |                                                                     
      | Place copyright information at the top of every subsystem in design.
      mask prompts: none "No parameters"
      mask help: Place copyright information at the top of every subsystem in design.
      mask Display:
      | NxtrConf = 'Nexteer Confidential';
      | 
      | sys = bdroot; %handle for the current model ("system")
      | first = get_param(sys,'Created');
      | first = first(end-3:end);  %year is last four digits
      | 
      | last = get_param(sys,'LastModifiedDate');
      | if isempty(last)
      |     last = datestr(now,'yyyy');
      | else
      |     last = last(end-3:end);
      | end
      | 
      | if strcmp(first,last)
      |     fprintf('%s -- Copyright %s Nexteer',NxtrConf,first)
      | else
      |     fprintf('%s -- %s%s- %s Nexteer',NxtrConf,char(169),first,last)
      | end
  Terminator : Terminator
  Out1 : Outport
  wires:
  Signal/1 -> Out1/1
  FltInjCon/1 -> Terminator/1

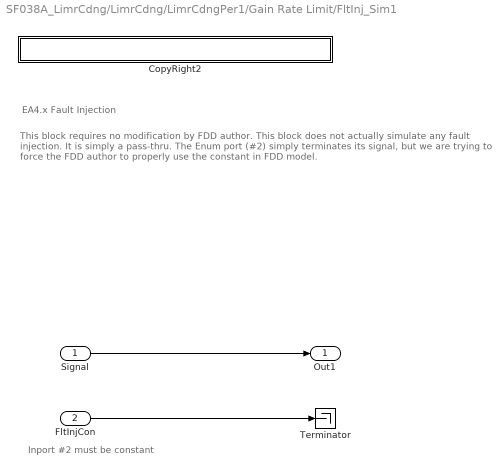
== system SF038A_LimrCdng/LimrCdng/LimrCdngPer1/Gain Rate Limit/FltInj_Sim1 ==
  note: This block requires no modification by FDD author.
      |
      | This block does not actually simulate any fault injection.  It is simply a pass-thru.
      |
      | The Enum port (#2) simply terminates its signal, but we are trying to force the FDD author
      | to properly use the constant in FDD model.
  note: EA4.x Fault Injection
  note: Inport #2 must be constant
  Signal : Inport
  FltInjCon : Inport  Port=2
  CopyRight2 : Subsystem  Description=|  mask(Copyright Information){none=on}
      | Copyright info block.                                               
      |                                                                     
      | Place copyright information at the top of every subsystem in design.
      mask prompts: none "No parameters"
      mask help: Place copyright information at the top of every subsystem in design.
      mask Display:
      | NxtrConf = 'Nexteer Confidential';
      | 
      | sys = bdroot; %handle for the current model ("system")
      | first = get_param(sys,'Created');
      | first = first(end-3:end);  %year is last four digits
      | 
      | last = get_param(sys,'LastModifiedDate');
      | if isempty(last)
      |     last = datestr(now,'yyyy');
      | else
      |     last = last(end-3:end);
      | end
      | 
      | if strcmp(first,last)
      |     fprintf('%s -- Copyright %s Nexteer',NxtrConf,first)
      | else
      |     fprintf('%s -- %s%s- %s Nexteer',NxtrConf,char(169),first,last)
      | end
  Terminator : Terminator
  Out1 : Outport
  wires:
  Signal/1 -> Out1/1
  FltInjCon/1 -> Terminator/1

== system SF038A_LimrCdng/LimrCdng/LimrCdngPer1/Torque Rate Limit/CopyRight2 ==

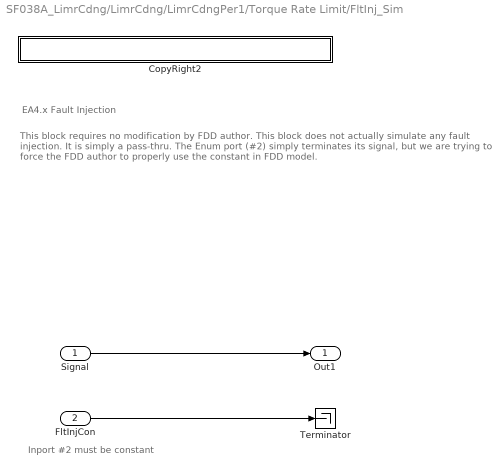
== system SF038A_LimrCdng/LimrCdng/LimrCdngPer1/Torque Rate Limit/FltInj_Sim ==
  note: This block requires no modification by FDD author.
      |
      | This block does not actually simulate any fault injection.  It is simply a pass-thru.
      |
      | The Enum port (#2) simply terminates its signal, but we are trying to force the FDD author
      | to properly use the constant in FDD model.
  note: EA4.x Fault Injection
  note: Inport #2 must be constant
  Signal : Inport
  FltInjCon : Inport  Port=2
  CopyRight2 : Subsystem  Description=|  mask(Copyright Information){none=on}
      | Copyright info block.                                               
      |                                                                     
      | Place copyright information at the top of every subsystem in design.
      mask prompts: none "No parameters"
      mask help: Place copyright information at the top of every subsystem in design.
      mask Display:
      | NxtrConf = 'Nexteer Confidential';
      | 
      | sys = bdroot; %handle for the current model ("system")
      | first = get_param(sys,'Created');
      | first = first(end-3:end);  %year is last four digits
      | 
      | last = get_param(sys,'LastModifiedDate');
      | if isempty(last)
      |     last = datestr(now,'yyyy');
      | else
      |     last = last(end-3:end);
      | end
      | 
      | if strcmp(first,last)
      |     fprintf('%s -- Copyright %s Nexteer',NxtrConf,first)
      | else
      |     fprintf('%s -- %s%s- %s Nexteer',NxtrConf,char(169),first,last)
      | end
  Terminator : Terminator
  Out1 : Outport
  wires:
  Signal/1 -> Out1/1
  FltInjCon/1 -> Terminator/1

== system SF038A_LimrCdng/LimrCdng/LimrCdngPer1/Gain Rate Limit/FltInj_Sim/CopyRight2 ==

== system SF038A_LimrCdng/LimrCdng/LimrCdngPer1/Gain Rate Limit/FltInj_Sim1/CopyRight2 ==

== system SF038A_LimrCdng/LimrCdng/LimrCdngPer1/Torque Rate Limit/FltInj_Sim/CopyRight2 ==
